simulink model "HIL_Testing_SW"  (Simulink 7.5)
settings: Solver=ode1  StartTime=0.0  StopTime=Inf  FixedStep=0.001  RelTol=1e-3
PostLoadFcn:
  | , if any(exist('dsrtsu_mdlpostloadfcn', 'file') == [2, 3, 6]), try dsrtsu_mdlpostloadfcn('Execute', bdroot); catch fprintf('Error in PostLoadFcn (dsrtsu_mdlpostloadfcn) for model "%s":\n %s\n', bdroot, lasterr); end, end,
undefined symbols (not defined in the file): CeBSER_Cnt_NumTempAxisPts, ChargeCord, ChargeCord_Control, ChargeToSOCCurr, ChrgCurrLim, CrntSens1Fine, CS_SOCSetPt, CyclerMaxChrgPwr, CyclerMaxDschrgPwr, deltaAhr, Drive_1, Drive_10, Drive_11, Drive_12, Drive_13, Drive_14, Drive_15, Drive_16, Drive_17, Drive_18, Drive_19, Drive_2, Drive_20, Drive_21, Drive_22, Drive_23, Drive_24, Drive_25, Drive_26, Drive_27, Drive_28, Drive_29, Drive_3, Drive_30, Drive_31, Drive_32, Drive_33, Drive_34, Drive_35, Drive_36, Drive_37, Drive_38, Drive_39, Drive_4, Drive_40, Drive_41, Drive_42, Drive_43, Drive_44, Drive_45, Drive_46, Drive_47, Drive_48, Drive_49, Drive_5, Drive_50, Drive_51, Drive_6, Drive_7, Drive_8 ... (+50)
libraries: simulink x129, rtican x50, rti2211sailib x5, rti2211serlib x5, rti2202miolib x3
(part 17 of 23)

== system HIL_Testing_SW/TX/Tx_Cycler/TX_ABC_ChB/msg_0x1A2_Upp_Lim_B_out ==
  Counter : Inport  OutDataType=sfix(16)  OutScaling=2^0
  Enable : EnablePort  StatesWhenEnabling=reset
  Constant1 : Constant  Value=1000  OutDataType=sfix(16)  OutScaling=2^0
  Data Store Read : DataStoreRead  DataStoreName=ChrgCurrLim  SampleTime=-1
  Data Store Read1 : DataStoreRead  DataStoreName=Voltage_Lid  SampleTime=-1
  Data Store Read2 : DataStoreRead  DataStoreName=CyclerMaxChrgPwr  SampleTime=-1
  Data Type Conversion : DataTypeConversion  OutDataTypeMode=double  OutDataType=fixdt(1, 16)  OutScaling=2^0  OutDataTypeStr=double
  Data Type Conversion1 : DataTypeConversion  OutDataTypeMode=double  OutDataType=fixdt(1, 16)  OutScaling=2^0  OutDataTypeStr=double
  Data Type Conversion{2..4,7} (4 alike) : DataTypeConversion  OutDataType=fixdt(1, 16)  OutScaling=2^0
  Product : Product  OutDataType=sfix(16)  OutScaling=2^0  RndMeth=Zero
  Terminator : Terminator
  Upp_Lim_B_out : rtican/RTICAN Transmit (TX)   SystemSampleTime=-1  Reserved1=[]  Reserved2=[]  Reserved3=[]  Reserved4=[]  SfcnMessage=[]  Msg_Struct=[]  BoardTypeNo=[]  BoardNo=[]  ChannelNo=[]  Parameters=[]  DialogFcn=[]  UnitName=[]  Revision=[]  UnitValues=[]  DSProperties=struct('RTI',struct('Version',uint32(5),'BlockType',struct('isSLSource',uint8(1),'isSLSink',uint8(1),'isHWSource',uint8(0),'isHWSink',uint8(0),'isSetup',uint8(0),'isInline',uint8(1),'isNonInline',uint8(0),'isInterrupt',uint8(0),'isChannelwise',uint8(0)),'IOBoardType','RTICAN','UnitType','MESSAGE','Identifier','TX','DialogType','MSVC','BlockSet','RTICAN','SlaveProcessor','CAN'))  RTIBlockInterface=struct('InputPortsWidth',int32([1 1 1 1]),'InputPortsActive',[1 1 1 1],'InputPortsName',{{'Upp_Powr_Lim_B_out','Counter_Stamp3_B','Upp_Curr_Lim_B_out','Upp_Volt_Lim_B_out'}},'InputPortsDataType',{{'SS_DOUBLE','SS_DOUBLE','SS_DOUBLE','SS_DOUBLE'}},'OutputPortsWidth',int32(1),'OutputPortsActive',1,'OutputPortsName',{{['TX status']}},'DialogFcn','rtican_message_interface_gui','BlockDisplay',{{'','center'}},'IconTransparency','on','InitLevel',3,'BlockName',struct('Token',{{'Upp_Lim_B_out'}}),'SampleTime',{{-1}},'TriggerPort',{{'none'}},'EnablePort',{{'none'}})  RTIBlockParameters=struct('BoardTypeNo',{{2211,'OFF',[]}},'BoardNo',{{2,'ON',[1 16]}},'ChannelNo',{{1,'ON',[1 2]}},'Parameters',{{struct('DataFileSupport',struct('DataFileSelectedMaster',1,'DataFileSelectedLocal',1,'DataFileName','c:\data\testing\av900_dbc\av900_mod.dbc|','DataFileDate',{{{['20-Apr-2011 08:23:37']}}},'SelectedFile','av900_dbc\av900_mod.dbc','InterfaceFcn','rtican_dbc_file_parser'),'Options',struct('StatusSelected',1,'TimeSelected',0,'DeltaTimeSelected',0,'DelayTimeSelected',0,'DelayTimeTXCommandSelected',0,'EncodeSetUnusedBitsToOne',0,'EnableMsgLoopback',0,'TriggerPort',struct('Selected',0,'TriggerType',0),'EnablePortSelected',0,'SignalOnPortnameSelected',1,'UserCoding',struct('Selected',0,'InterfaceFile','UserEncodingFile','FcnName','UserEncodeFcn','InportSelected',0,'InportWidth',1,'OutportSelected',0,'OutportWidth',1),'TerminationMsg',struct('Selected',0,'Byte0_7','0'),'InitialMsg',struct('Selected',0,'Byte0_7','0')),'Message',struct('MsgOnBlocknameSelected',1,'MsgName','Upp_Lim_B_out','MsgIdFormat',0,'MsgId',418,'MsgLength',7,'NumSignals',4,'SampleTime',-1,'StartTime',struct('Selected',0,'Value',0),'AutoRepeatTime',struct('Selected',0,'Value',0.1),'Timeout',struct('Selected',0,'Value',0.1),'DelayTime',struct('Selected',0,'Value',0.1),'Signal',struct('SgnName',{'Upp_Powr_Lim_B_out','Counter_Stamp3_B','Upp_Curr_Lim_B_out','Upp_Volt_Lim_B_out'},'SgnStartBit',{0,0,16,32},'SgnLength',{16,8,16,16},'SgnType',{0,0,0,0},'ModeValue',{-1,-1,-1,-1},'DataType',{1,0,1,1},'ByteLayout',{2,0,2,2},'Factor',{10,1,0.04,0.05},'Offset',{0,0,0,0},'SgnComment',{{''},{''},{''},{''}},'SgnUnit',{'W','code','A','V'},'Min',{-327680,0,-1310.72,-1638.4},'Max',{327670,255,1310.68,1638.35},'SLDataType',{'SS_DOUBLE','SS_DOUBLE','SS_DOUBLE','SS_DOUBLE'}),'MsgIdNumFormat',0,'MsgComment',{{''}}),'Version',1.2,'general',struct('isFromLib',0)),'OFF',[]}},'GroupId',{{struct('Group',{{'RTICAN'}},'No',6,'Behavior',{{'NAMECHANGE'}},'BlockType',{{'SINK'}},'NameChangeFlag',0),'OFF',[]}},'SFcnRTICANMessage',{{struct('MsgType','TX','SFcnPortType','Scalar','MsgName','Upp_Lim_B_out','MsgIdFormat','STD','MsgId',418,'MsgLength',7,'NumSignals',4,'SampleTime',-1,'StartTime',struct('Selected','no','Value',0),'AutoRepeatTime',struct('Selected','no','Value',0.1),'Timeout',struct('Selected','no','Value',0.1),'Signal',struct('SgnName',{'Upp_Powr_Lim_B_out','Counter_Stamp3_B','Upp_Curr_Lim_B_out','Upp_Volt_Lim_B_out'},'SgnStartBit',{0,0,16,32},'SgnLength',{16,8,16,16},'SgnType',{'standard','standard','standard','standard'},'ModeValue',{-1,-1,-1,-1},'DataType',{['signed int'],['unsigned int'],['signed int'],['signed int']},'ByteLayout',{['motorola back.'],['little endian'],['motorola back.'],['motorola back.']},'Factor',{10,1,0.04,0.05},'Offset',{0,0,0,0},'SLDataType',{'SS_DOUBLE','SS_DOUBLE','SS_DOUBLE','SS_DOUBLE'}),'StatusSelected','yes','TimeSelected','no','DeltaTimeSelected','no','DelayTimeSelected','no','DelayTimeTXCommandSelected','no','EncodeSetUnusedBitsToOne','no','EnableMsgLoopback','no','TriggerPort',struct('Selected','no','TriggerType',0),'EnablePortSelected','no','UserCoding',struct('Selected','no','InterfaceFile','UserEncodingFile','FcnName','UserEncodeFcn','InportSelected','no','InportWidth',1,'OutportSelected','no','OutportWidth',1),'TerminationMsg',struct('Selected','no','Byte0','0x00','Byte1','0x00','Byte2','0x00','Byte3','0x00','Byte4','0x00','Byte5','0x00','Byte6','0x00','Byte7','0x00'),'InitialMsg',struct('Selected','no','Byte0','0x00','Byte1','0x00','Byte2','0x00','Byte3','0x00','Byte4','0x00','Byte5','0x00','Byte6','0x00','Byte7','0x00'),'BoardType','DS2211','BoardNo',2,'ControllerNo',1),'OFF',[]}},'TLCFileName',{{'rtican_tx_message','OFF',[]}})  RTISFcnParameters=struct('SFcnRTICANMessage','struct','TLCFileName','char')  RTIBlockParaDefault=struct('BoardTypeNo',4302,'BoardNo',1,'ChannelNo',1,'Parameters',struct('DataFileSupport',struct('DataFileSelectedMaster',0,'DataFileSelectedLocal',0,'DataFileName','','DataFileDate','','SelectedFile',['<no file selected>']),'Options',struct('StatusSelected',1,'TimeSelected',1,'DeltaTimeSelected',1,'DelayTimeSelected',1,'DelayTimeTXCommandSelected',0,'EncodeSetUnusedBitsToOne',0,'EnableMsgLoopback',0,'TriggerPort',struct('Selected',0,'TriggerType','rising'),'EnablePortSelected',0,'SignalOnPortnameSelected',1,'UserCoding',struct('Selected',0,'InterfaceFile','UserEncodingFile','FcnName','UserEncodeFcn','InportSelected',0,'InportWidth',1,'OutportSelected',0,'OutportWidth',1),'TerminationMsg',struct('Selected',0,'Byte0_7','0'),'InitialMsg',struct('Selected',0,'Byte0_7','0')),'Message',struct('MsgOnBlocknameSelected',0,'MsgName',['TX Message'],'MsgIdFormat',0,'MsgId',100,'MsgLength',8,'NumSignals',1,'SampleTime',-1,'StartTime',struct('Selected',0,'Value',0),'AutoRepeatTime',struct('Selected',0,'Value',0.1),'Timeout',struct('Selected',0,'Value',0.1),'DelayTime',struct('Selected',0,'Value',0.1),'Signal',struct('SgnName',['TX signal'],'SgnStartBit',0,'SgnLength',8,'SgnType',0,'ModeValue',-1,'DataType',0,'SLDataType','SS_DOUBLE','ByteLayout',0,'Factor',1,'Offset',0,'Min',0,'Max',255,'SgnComment',{{}},'SgnUnit',''),'MsgIdNumFormat',0,'MsgComment',{{''}}),'Version',1.2,'general',struct('isFromLib',1)),'GroupId',struct('Group',{{'RTICAN'}},'No',1,'Behavior',{{'NAMECHANGE'}},'BlockType',{{'SINK'}},'NameChangeFlag',0),'SFcnRTICANMessage',struct('MsgType','TX','MsgName',['TX Message'],'MsgIdFormat','STD','MsgId',100,'MsgLength',2,'NumSignals',1,'SampleTime',-1,'StartTime',struct('Selected','no','Value',0),'AutoRepeatTime',struct('Selected','no','Value',0.1),'Timeout',struct('Selected','no','Value',0.1),'DelayTime',struct('Selected','no','Value',0.1),'Signal',struct('SgnName',['TX signal'],'SgnStartBit',0,'SgnLength',8,'SgnType','standard','ModeValue',-1,'DataType',['unsigned int'],'ByteLayout',['little endian'],'SLDataType','SS_DOUBLE','Factor',1,'Offset',0),'StatusSelected','yes','TimeSelected','yes','DeltaTimeSelected','yes','DelayTimeSelected','yes','EnablePortSelected','no','EnableMsgLoopback','no','DelayTimeTXCommandSelected','no','EncodeSetUnusedBitsToOne','no','UserCoding',struct('Selected','no','InterfaceFile','UserDecodingFile','FcnName','UserDecodeFcn','InportSelected','no','InportWidth',1,'OutportSelected','no','OutportWidth',1),'TerminationMsg',struct('Selected','no','Byte0','0x00','Byte1','0x00','Byte2','0x00','Byte3','0x00','Byte4','0x00','Byte5','0x00','Byte6','0x00','Byte7','0x00'),'InitialMsg',struct('Selected','no','Byte0','0x00','Byte1','0x00','Byte2','0x00','Byte3','0x00','Byte4','0x00','Byte5','0x00','Byte6','0x00','Byte7','0x00'),'TriggerPort',struct('Selected','no','TriggerType','rising'),'BoardType','DS4302','BoardNo',1,'ControllerNo',1,'SFcnPortType','Scalar'),'TLCFileName','rtican_tx_message')
      settings: AttributesFormatString=Group Id: RTICAN6\n
  wires:
  Data Store Read/1 -> Data Type Conversion/1
  Data Store Read1/1 -> Data Type Conversion1/1
  Data Store Read2/1 -> Product/1
  Constant1/1 -> Product/2
  Upp_Lim_B_out/1 -> Terminator/1
  Data Type Conversion1/1 -> Data Type Conversion4/1
  Data Type Conversion/1 -> Data Type Conversion3/1
  Counter/1 -> Data Type Conversion2/1
  Product/1 -> Data Type Conversion7/1
  Data Type Conversion7/1 -> Upp_Lim_B_out/1
  Data Type Conversion2/1 -> Upp_Lim_B_out/2
  Data Type Conversion3/1 -> Upp_Lim_B_out/3
  Data Type Conversion4/1 -> Upp_Lim_B_out/4

== system HIL_Testing_SW/HWO/TX HVEM/ChargeCord_Control/Cord Connected/110 Connected ==
  note: Updated to 108 cals for Ofst and Slp
  Volt_in : Inport  OutDataType=sfix(16)  OutScaling=2^0
  Current_in : Inport  Port=2  OutDataType=sfix(16)  OutScaling=2^0
  Temp_in : Inport  Port=3  OutDataType=sfix(16)  OutScaling=2^0
  DC_in : Inport  Port=4  OutDataType=sfix(16)  OutScaling=2^0
  Action Port : ActionPort  ActionType=then
  110_Volts : Constant  Value=110  OutDataType=sfix(16)  OutScaling=2^0  OutDataTypeStr=Inherit: Inherit via back propagation
  Fcn : Fcn  Expr=((u(1)-32.5)/2.75)
  Volt_out : Outport  OutDataType=sfix(16)  OutScaling=2^0
  Current_out : Outport  Port=2  OutDataType=sfix(16)  OutScaling=2^0
  Temp_out : Outport  Port=3  OutDataType=sfix(16)  OutScaling=2^0
  DC_Out : Outport  Port=4  OutDataType=sfix(16)  OutScaling=2^0
  PrcsdVolt_DC : Outport  Port=5  OutDataType=sfix(16)  OutScaling=2^0
  wires:
  DC_in/1 -> DC_Out/1
  Temp_in/1 -> Temp_out/1
  Current_in/1 -> Current_out/1
  Fcn/1 -> PrcsdVolt_DC/1
  Volt_in/1 -> Volt_out/1
  110_Volts/1 -> Fcn/1

== system HIL_Testing_SW/HWO/TX HVEM/ChargeCord_Control/Cord Connected/220 Connected ==
  note: Updated to 108 cals for Ofst and Slp
  Volt_in : Inport  OutDataType=sfix(16)  OutScaling=2^0
  Current_in : Inport  Port=2  OutDataType=sfix(16)  OutScaling=2^0
  Temp_in : Inport  Port=3  OutDataType=sfix(16)  OutScaling=2^0
  DC_in : Inport  Port=4  OutDataType=sfix(16)  OutScaling=2^0
  Action Port : ActionPort  ActionType=elseif
  220_Volts : Constant  Value=220  OutDataType=sfix(16)  OutScaling=2^0  OutDataTypeStr=Inherit: Inherit via back propagation
  Fcn : Fcn  Expr=((u(1)-32.5)/2.75)
  Volt_out : Outport  OutDataType=sfix(16)  OutScaling=2^0
  Current_out : Outport  Port=2  OutDataType=sfix(16)  OutScaling=2^0
  Temp_out : Outport  Port=3  OutDataType=sfix(16)  OutScaling=2^0
  DC_Out : Outport  Port=4  OutDataType=sfix(16)  OutScaling=2^0
  PrcsdVolt_DC : Outport  Port=5  OutDataType=sfix(16)  OutScaling=2^0
  wires:
  Volt_in/1 -> Volt_out/1
  Current_in/1 -> Current_out/1
  Temp_in/1 -> Temp_out/1
  DC_in/1 -> DC_Out/1
  Fcn/1 -> PrcsdVolt_DC/1
  220_Volts/1 -> Fcn/1

== system HIL_Testing_SW/HWO/TX HVEM/ChargeCord_Control/Cord Connected/AC Enabled ==
  Volt_in : Inport  OutDataType=sfix(16)  OutScaling=2^0
  Current_in : Inport  Port=2  OutDataType=sfix(16)  OutScaling=2^0
  Action Port : ActionPort  ActionType=then
  Volt_out : Outport  OutDataType=sfix(16)  OutScaling=2^0
  Current_out : Outport  Port=2  OutDataType=sfix(16)  OutScaling=2^0
  wires:
  Current_in/1 -> Current_out/1
  Volt_in/1 -> Volt_out/1

== system HIL_Testing_SW/HWO/TX HVEM/ChargeCord_Control/Cord Connected/AC Not Enabled ==
  Volt_in : Inport  OutDataType=sfix(16)  OutScaling=2^0
  Current_in : Inport  Port=2  OutDataType=sfix(16)  OutScaling=2^0
  Action Port : ActionPort  ActionType=else
  Volt_out : Outport  OutDataType=sfix(16)  OutScaling=2^0
  Current_out : Outport  Port=2  OutDataType=sfix(16)  OutScaling=2^0
  wires:
  Volt_in/1 -> Volt_out/1
  Current_in/1 -> Current_out/1

== system HIL_Testing_SW/HWO/TX HVEM/ChargeCord_Control/Cord Connected/Not Connected ==
  Volt_in : Inport  OutDataType=sfix(16)  OutScaling=2^0
  Current_in : Inport  Port=2  OutDataType=sfix(16)  OutScaling=2^0
  Temp_in : Inport  Port=3  OutDataType=sfix(16)  OutScaling=2^0
  DC_in : Inport  Port=4  OutDataType=sfix(16)  OutScaling=2^0
  Action Port : ActionPort  ActionType=else
  NotConnected_Volts : Constant  Value=100  OutDataType=sfix(16)  OutScaling=2^0  OutDataTypeStr=Inherit: Inherit via back propagation
  Volt_out : Outport  OutDataType=sfix(16)  OutScaling=2^0
  Current_out : Outport  Port=2  OutDataType=sfix(16)  OutScaling=2^0
  Temp_out : Outport  Port=3  OutDataType=sfix(16)  OutScaling=2^0
  DC_Out : Outport  Port=4  OutDataType=sfix(16)  OutScaling=2^0
  PrcsdVolt_DC : Outport  Port=5  OutDataType=sfix(16)  OutScaling=2^0
  wires:
  Volt_in/1 -> Volt_out/1
  Current_in/1 -> Current_out/1
  Temp_in/1 -> Temp_out/1
  DC_in/1 -> DC_Out/1
  NotConnected_Volts/1 -> PrcsdVolt_DC/1

== system HIL_Testing_SW/LionsHeart/FeaturePresentation/Down_to_Business/DriveProfile_ModeControl/Capacity Test ==
  Current_Cntrl : Inport  OutDataType=fixdt(1, 16)  OutScaling=2^0
  Voltage_Cntrl : Inport  Port=2  OutDataType=fixdt(1, 16)  OutScaling=2^0
  MaxCall_PackVolt : Inport  Port=3  OutDataType=fixdt(1, 16)  OutScaling=2^0
  MinCall_PackVolt : Inport  Port=4  OutDataType=fixdt(1, 16)  OutScaling=2^0
  CyclerVoltage : Inport  Port=5  OutDataType=fixdt(1, 16)  OutScaling=2^0
  Enable : EnablePort  StatesWhenEnabling=reset
  Capacity_Test : Stateflow chart  TreatAsAtomicUnit=on
  Data Store Read : DataStoreRead  DataStoreName=Voltage_Floor  SampleTime=0
  Data Store Read1 : DataStoreRead  DataStoreName=Voltage_Lid  SampleTime=0
  Data Store Read10 : DataStoreRead  DataStoreName=DschrgCurrLim  SampleTime=0
  Data Store Read11 : DataStoreRead  DataStoreName=CapCycles  SampleTime=0
  Data Store Read12 : DataStoreRead  DataStoreName=CapRestTime  SampleTime=0
  Data Store Read13 : DataStoreRead  DataStoreName=OCV_Zero  SampleTime=0
  Data Store Read2 : DataStoreRead  DataStoreName=TerminationCurrent  SampleTime=0
  Data Store Read3 : DataStoreRead  DataStoreName=Voltage_Floor_Cell  SampleTime=0
  Data Store Read4 : DataStoreRead  DataStoreName=C_Rate  SampleTime=0
  Data Store Read5 : DataStoreRead  DataStoreName=Voltage_Lid_Cell  SampleTime=0
  Data Store Read6 : DataStoreRead  DataStoreName=RateFactor  SampleTime=0
  Data Store Read7 : DataStoreRead  DataStoreName=MaxCell_Enbl  SampleTime=0
  Data Store Read8 : DataStoreRead  DataStoreName=MinCell_Enbl  SampleTime=0
  Data Store Read9 : DataStoreRead  DataStoreName=ChrgCurrLim  SampleTime=0
  Data Store Write1 : DataStoreWrite  DataStoreName=ChrgCurrLim  SampleTime=-1
  Data Store Write2 : DataStoreWrite  DataStoreName=DschrgCurrLim  SampleTime=-1
  Data Store Write3 : DataStoreWrite  DataStoreName=ContactorOverride  SampleTime=-1
  Data Type Conversion : DataTypeConversion  OutDataTypeMode=single  OutDataType=sfix(16)  OutScaling=2^0  OutDataTypeStr=single
  Data Type Conversion1 : DataTypeConversion  OutDataTypeMode=single  OutDataType=sfix(16)  OutScaling=2^0  OutDataTypeStr=single
  Gain : Gain  ParameterDataType=fixdt(1, 16)  ParameterScaling=2^0  OutDataType=fixdt(1, 16)  OutScaling=2^0
  Terminator1 : Terminator
  Terminator2 : Terminator
  Terminator4 : Terminator
  simstep : Constant  Tag=R12-1  Value=SimStep_dT  OutDataTypeMode=double  OutDataType=sfix(16)  OutScaling=2^0  OutDataTypeStr=double
  Profile_Data_cap : Outport  OutDataType=sfix(16)  OutScaling=2^0
  Mode_Cntrl_cap : Outport  Port=2  OutDataType=sfix(16)  OutScaling=2^0
  CapStep : Outport  Port=3  OutDataType=sfix(16)  OutScaling=2^0
  ResetSOCFlg : Outport  Port=4  OutDataType=sfix(16)  OutScaling=2^0
  wires:
  Current_Cntrl/1 -> [Current_Cntrl]
  Voltage_Cntrl/1 -> [Voltage_Cntrl]
  simstep/1 -> Data Type Conversion1/1
  Data Type Conversion/1 -> Profile_Data_cap/1
  Capacity_Test/1(Control_Value_cap) -> Data Type Conversion/1
  Data Type Conversion1/1 -> Capacity_Test/7(sim_step_time)
  Capacity_Test/2(WaitTime) -> Terminator2/1  "Waitime"
  Capacity_Test/4(cycle) -> Terminator4/1  "cycle"
  Data Store Read9/1 -> Capacity_Test/9(ChrgCurrLim)
  Data Store Read10/1 -> Capacity_Test/10(DischrgCurrLim)
  Capacity_Test/5(DischrgCurrLim_Tmp) -> Data Store Write2/1
  Capacity_Test/6(ChrgCurrLim_Tmp) -> Data Store Write1/1
  Capacity_Test/7(Step) -> CapStep/1
  MaxCall_PackVolt/1 -> [MaxCell_PackVolt]
  MinCall_PackVolt/1 -> [MinCell_PackVolt]
  [MinCell_PackVolt] -> Capacity_Test/11(PackVolt_MinCell)
  [MaxCell_PackVolt] -> Capacity_Test/12(PackVolt_MaxCell)
  Data Store Read6/1 -> Capacity_Test/13(RateFactor)
  Capacity_Test/3(Mode_Cntrl_cap) -> Mode_Cntrl_cap/1
  Data Store Read3/1 -> Capacity_Test/14(Vfloor_cell)
  Data Store Read5/1 -> Capacity_Test/15(Vlid_cell)
  Data Store Read7/1 -> Capacity_Test/16(MaxCell_Enbl)
  Data Store Read8/1 -> Capacity_Test/17(MinCell_Enbl)
  CyclerVoltage/1 -> [CyclerVoltage]
  [CyclerVoltage] -> Capacity_Test/18(CyclerVoltage)
  Data Store Read11/1 -> Capacity_Test/6(NumberCycles)
  Data Store Read12/1 -> Capacity_Test/8(RestTime)
  Data Store Read4/1 -> Capacity_Test/20(CRate)
  [Voltage_Cntrl] -> Capacity_Test/4(Voltage_Cntrl)
  [Current_Cntrl] -> Capacity_Test/5(Current_Cntrl)
  Data Store Read1/1 -> Capacity_Test/2(Vlid)
  Data Store Read2/1 -> Capacity_Test/3(CurrentTerm)
  Data Store Read13/1 -> Capacity_Test/19(OCV_Zero)
  Capacity_Test/8(ContactorOverride) -> Data Store Write3/1
  Gain/1 -> Terminator1/1  "Cappy2"
  Capacity_Test/9(Cappy) -> Gain/1  "Cappy"
  Data Store Read/1 -> Capacity_Test/1(Vfloor)
  Capacity_Test/10(ResetSOCFlg) -> ResetSOCFlg/1  "ResetSOCFlg"

== system HIL_Testing_SW/LionsHeart/FeaturePresentation/Down_to_Business/DriveProfile_ModeControl/Charging_Mode ==
  note: Select Current for Charge
  Current : Inport  OutDataType=fixdt(1, 16)  OutScaling=2^0
  Voltage : Inport  Port=2  OutDataType=fixdt(1, 16)  OutScaling=2^0
  ChargeCurrSelect : Inport  Port=3  OutDataType=fixdt(1, 16)  OutScaling=2^0
  SOCTarget : Inport  Port=4  OutDataType=fixdt(1, 16)  OutScaling=2^0
  PackVolt_MaxCell : Inport  Port=5  OutDataType=fixdt(1, 16)  OutScaling=2^0
  PackVolt_MinCell : Inport  Port=6  OutDataType=fixdt(1, 16)  OutScaling=2^0
  SOC : Inport  Port=7  OutDataType=fixdt(1, 16)  OutScaling=2^0
  Voltage_Cntrl : Inport  Port=8  OutDataType=fixdt(1, 16)  OutScaling=2^0
  Current_Cntrl : Inport  Port=9  OutDataType=fixdt(1, 16)  OutScaling=2^0
  Enable : EnablePort  StatesWhenEnabling=reset
  Charge Selector : MultiPortSwitch  DataPortOrder=Zero-based contiguous  zeroidx=on  OutDataType=sfix(16)  OutScaling=2^0
  Charging Logic1 : Stateflow chart  TreatAsAtomicUnit=on
  Data Store Read : DataStoreRead  DataStoreName=VoltageTerm  SampleTime=0
  Data Store Read1 : DataStoreRead  DataStoreName=TerminationCurrent  SampleTime=0
  Data Store Read10 : DataStoreRead  DataStoreName=DschrgCurrLim  SampleTime=0
  Data Store Read11 : DataStoreRead  DataStoreName=RateFactor  SampleTime=0
  Data Store Read12 : DataStoreRead  DataStoreName=Voltage_Floor  SampleTime=0
  Data Store Read13 : DataStoreRead  DataStoreName=CyclerOffset  SampleTime=0
  Data Store Read15 : DataStoreRead  DataStoreName=ChargeToSOCRate  SampleTime=0
  Data Store Read2 : DataStoreRead  DataStoreName=WaitTime  SampleTime=0
  Data Store Read3 : DataStoreRead  DataStoreName=Voltage_Lid  SampleTime=0
  Data Store Read4 : DataStoreRead  DataStoreName=MaxCell_Enbl  SampleTime=0
  Data Store Read5 : DataStoreRead  DataStoreName=VoltageTerm_MaxCell  SampleTime=0
  Data Store Read6 : DataStoreRead  DataStoreName=TwoTwentyChrgCurr  SampleTime=0
  Data Store Read7 : DataStoreRead  DataStoreName=OneTenChargeCurr  SampleTime=0
  Data Store Read8 : DataStoreRead  DataStoreName=MinCell_Enbl  SampleTime=0
  Data Store Read9 : DataStoreRead  DataStoreName=ChrgCurrLim  SampleTime=0
  Data Store Write15 : DataStoreWrite  DataStoreName=ChrgCurrLim  SampleTime=-1
  Data Store Write16 : DataStoreWrite  DataStoreName=DschrgCurrLim  SampleTime=-1
  Data Type Conversion : DataTypeConversion  OutDataTypeMode=single  OutDataType=sfix(16)  OutScaling=2^0  OutDataTypeStr=single
  Data Type Conversion1 : DataTypeConversion  OutDataTypeMode=single  OutDataType=sfix(16)  OutScaling=2^0  OutDataTypeStr=single
  Terminator : Terminator
  simstep : Constant  Tag=R12-1  Value=SimStep_dT  OutDataTypeMode=double  OutDataType=sfix(16)  OutScaling=2^0  OutDataTypeStr=double
  Profile_Data_chrg : Outport  OutDataType=sfix(16)  OutScaling=2^0
  Mode_Cntrl_chrg : Outport  Port=2  OutDataType=sfix(16)  OutScaling=2^0
  ChargeStep : Outport  Port=3  OutDataType=sfix(16)  OutScaling=2^0
  wires:
  Charge Selector/1 -> [ChargeCurrent]
  Current/1 -> [CyclerCurrent]
  Voltage/1 -> [Voltage]
  [ChargeCurrent] -> Charging Logic1/1(RateChrg)
  simstep/1 -> Data Type Conversion1/1
  Data Type Conversion1/1 -> Charging Logic1/5(sim_step_time)
  Data Store Read2/1 -> Charging Logic1/6(WaitTime1)
  SOC/1 -> Charging Logic1/8(SOC)
  [ChargeCurrSelect] -> Charging Logic1/7(ChargeSelect)
  Charging Logic1/3(Mode_Cntrl_cap) -> Mode_Cntrl_chrg/1
  Charging Logic1/1(Control_Value_cap) -> Data Type Conversion/1
  Charging Logic1/2(WaitTime) -> Terminator/1
  Data Store Read1/1 -> Charging Logic1/3(CurrentTerm)
  Data Store Read3/1 -> Charging Logic1/9(VoltageLid)
  Data Store Read6/1 -> Charge Selector/3
  Data Store Read7/1 -> Charge Selector/2
  Charging Logic1/4(ChargeLimit_Temp) -> Data Store Write15/1
  Charging Logic1/5(DisChrgCurr_Limit) -> Data Store Write16/1
  Data Store Read9/1 -> Charging Logic1/10(ChargeLimitCal)
  Data Store Read10/1 -> Charging Logic1/11(DisChrgCurrLimit_Cal)
  Charging Logic1/6(Step) -> ChargeStep/1
  ChargeCurrSelect/1 -> [ChargeCurrSelect]
  [ChargeCurrSelect] -> Charge Selector/1
  [Current_Cntrl] -> Charging Logic1/4(Current_Cntrl)
  [Voltage] -> Charging Logic1/12(CyclerVoltage)
  Data Store Read11/1 -> Charging Logic1/14(RateFactor)
  Data Type Conversion/1 -> Profile_Data_chrg/1
  [SOCTarget] -> Charging Logic1/13(SOCTarget)
  Data Store Read/1 -> Charging Logic1/2(VoltageSetPoint)
  SOCTarget/1 -> [SOCTarget]
  Data Store Read12/1 -> Charging Logic1/15(VFloor)
  PackVolt_MaxCell/1 -> [PackVoltage_MaxCell]
  PackVolt_MinCell/1 -> [PackVoltage_MinCell]
  [PackVoltage_MaxCell] -> Charging Logic1/16(PackVoltage_MaxCell)
  [PackVoltage_MinCell] -> Charging Logic1/17(PackVoltage_MinCell)
  Data Store Read5/1 -> Charging Logic1/18(VoltageSetPt_Max)
  Data Store Read15/1 -> Charge Selector/4
  Data Store Read4/1 -> Charging Logic1/20(MaxCell_Enbl)
  Data Store Read8/1 -> Charging Logic1/21(MinCell_Enbl)
  Voltage_Cntrl/1 -> [Voltage_Cntrl]
  Current_Cntrl/1 -> [Current_Cntrl]
  [Voltage_Cntrl] -> Charging Logic1/19(Voltage_Cntrl)
  Data Store Read13/1 -> Charging Logic1/22(CyclerOffset)

== system HIL_Testing_SW/LionsHeart/FeaturePresentation/Down_to_Business/DriveProfile_ModeControl/Drive_Profile ==
  note: Mode_Cntrl:
      | ****************
      | 0 = Voltage
      | 1 = Current
      | 2 = Power
      | 3 = Standby
  cycle_enable : Inport  OutDataType=sfix(16)  OutScaling=2^0
  SOC : Inport  Port=2  OutDataType=sfix(16)  OutScaling=2^0
  Current : Inport  Port=3  OutDataType=fixdt(1, 16)  OutScaling=2^0
  Voltage : Inport  Port=4  OutDataType=fixdt(1, 16)  OutScaling=2^0
  BatTemp : Inport  Port=5  OutDataType=fixdt(1, 16)  OutScaling=2^0
  PowerCycle : Inport  Port=6  OutDataType=sfix(16)  OutScaling=2^0
  CSSwitch : Inport  Port=7  OutDataType=sfix(16)  OutScaling=2^0
  StartTime : Inport  Port=8  OutDataType=sfix(16)  OutScaling=2^0
  EndTime : Inport  Port=9  OutDataType=sfix(16)  OutScaling=2^0
  Enable : EnablePort  StatesWhenEnabling=reset
  CD : Subsystem
  Data Type Conversion1 : DataTypeConversion  OutDataTypeMode=boolean  OutDataType=sfix(16)  OutScaling=2^0  OutDataTypeStr=boolean
  PowerMode : Constant  Value=single(2)  OutDataType=sfix(16)  OutScaling=2^0
  Relational Operator : RelationalOperator  LogicOutDataTypeMode=boolean  OutDataTypeStr=boolean
  Standby : Constant  Value=single(3)  OutDataType=sfix(16)  OutScaling=2^0
  Switch : Switch  Threshold=.5  OutDataType=sfix(16)  OutScaling=2^0
  Profile_Data_drive : Outport  OutDataType=sfix(16)  OutScaling=2^0
  Mode_Cntrl_drive : Outport  Port=2  OutDataType=sfix(16)  OutScaling=2^0
  ProfileEndTime : Outport  Port=3  OutDataType=sfix(16)  OutScaling=2^0
  LoopTime : Outport  Port=4  OutDataType=sfix(16)  OutScaling=2^0
  wires:
  SOC/1 -> [SOC]
  BatTemp/1 -> [BatTemp]
  Voltage/1 -> [Voltage]
  Current/1 -> [Current]
  cycle_enable/1 -> Data Type Conversion1/1
  PowerCycle/1 -> [Power_Cycle]
  PowerMode/1 -> Switch/3
  Switch/1 -> Mode_Cntrl_drive/1
  [Loop_Time] -> Relational Operator/1
  [ProfileEndTime] -> Relational Operator/2
  Relational Operator/1 -> Switch/2
  Standby/1 -> Switch/1
  CSSwitch/1 -> [SwitchMode]
  CD/2(LoopTime) -> [Loop_TimeCD]
  CD/1(ProfileTrigger) -> [ProfileData_PowerCD]
  [Power_Cycle] -> CD/1(PowercyleSelect)
  CD/3(ProfileEndTime) -> [ProfileEndTimeCD]
  Data Type Conversion1/1 -> [CycleEnable]
  [CycleEnable] -> CD/2(cycleEnbl)
  [ProfileData_PowerCD] -> Profile_Data_drive/1
  [Loop_TimeCD] -> LoopTime/1, [Loop_Time]
  [ProfileEndTimeCD] -> ProfileEndTime/1, [ProfileEndTime]
  StartTime/1 -> CD/3(StartTime)
  EndTime/1 -> CD/4(EndTime)

== system HIL_Testing_SW/LionsHeart/FeaturePresentation/Down_to_Business/DriveProfile_ModeControl/HPPC Test ==
  Current : Inport  OutDataType=fixdt(1, 16)  OutScaling=2^0
  Voltage : Inport  Port=2  OutDataType=fixdt(1, 16)  OutScaling=2^0
  Enable : EnablePort  StatesWhenEnabling=reset
  BeforeTime : Constant  Value=60  OutDataTypeMode=single  OutDataType=fixdt(1, 16)  OutScaling=2^0  OutDataTypeStr=single
  BtwnTime : Constant  Value=40  OutDataTypeMode=single  OutDataType=fixdt(1, 16)  OutScaling=2^0  OutDataTypeStr=single
  ChargeRate : Constant  OutDataTypeMode=single  OutDataType=fixdt(1, 16)  OutScaling=2^0  OutDataTypeStr=single
  Data Store Read : DataStoreRead  DataStoreName=VoltageTerm  SampleTime=0
  Data Store Read1 : DataStoreRead  DataStoreName=Voltage_Floor  SampleTime=0
  Data Store Read2 : DataStoreRead  DataStoreName=TerminationCurrent  SampleTime=0
  Data Store Read4 : DataStoreRead  DataStoreName=PackCapacity  SampleTime=0
  Data Store Read9 : DataStoreRead  DataStoreName=ChrgCurrLim  SampleTime=0
  Data Store Write15 : DataStoreWrite  DataStoreName=ChrgCurrLim  SampleTime=-1
  Data Type Conversion : DataTypeConversion  OutDataTypeMode=single  OutDataType=sfix(16)  OutScaling=2^0  OutDataTypeStr=single
  Data Type Conversion4 : DataTypeConversion  OutDataTypeMode=single  OutDataType=sfix(16)  OutScaling=2^0  OutDataTypeStr=single
  DischrgRate : Constant  Value=-1  OutDataTypeMode=single  OutDataType=fixdt(1, 16)  OutScaling=2^0  OutDataTypeStr=single
  FirstDischgTime : Constant  Value=150  OutDataTypeMode=single  OutDataType=fixdt(1, 16)  OutScaling=2^0  OutDataTypeStr=single
  HPPC_Test : Stateflow chart  TreatAsAtomicUnit=on
  PlchgCurr : Constant  Value=225  OutDataTypeMode=single  OutDataType=fixdt(1, 16)  OutScaling=2^0  OutDataTypeStr=single
  PldschgCurr : Constant  Value=-400  OutDataTypeMode=single  OutDataType=fixdt(1, 16)  OutScaling=2^0  OutDataTypeStr=single
  Product2 : Product  OutDataType=fixdt(1, 16)  OutScaling=2^0  RndMeth=Zero
  Product3 : Product  OutDataType=fixdt(1, 16)  OutScaling=2^0  RndMeth=Zero
  PulseTime : Constant  Value=10  OutDataTypeMode=single  OutDataType=fixdt(1, 16)  OutScaling=2^0  OutDataTypeStr=single
  RemDschgTime : Constant  Value=150  OutDataTypeMode=single  OutDataType=fixdt(1, 16)  OutScaling=2^0  OutDataTypeStr=single
  Rest : Constant  Value=7200  OutDataTypeMode=single  OutDataType=fixdt(1, 16)  OutScaling=2^0  OutDataTypeStr=single
  RestLong : Constant  Value=18000  OutDataTypeMode=single  OutDataType=fixdt(1, 16)  OutScaling=2^0  OutDataTypeStr=single
  RestShort : Constant  Value=60  OutDataTypeMode=single  OutDataType=fixdt(1, 16)  OutScaling=2^0  OutDataTypeStr=single
  Terminator : Terminator
  simstep : Constant  Tag=R12-1  Value=SimStep_dT  OutDataTypeMode=double  OutDataType=sfix(16)  OutScaling=2^0  OutDataTypeStr=double
  Mode_Cntrl_HPPC : Outport  OutDataType=sfix(16)  OutScaling=2^0
  Profile_Data_HPPC : Outport  Port=2  OutDataType=sfix(16)  OutScaling=2^0
  wires:
  Current/1 -> [Current]
  Voltage/1 -> [Voltage]
  ChargeRate/1 -> Product2/1
  Data Store Read4/1 -> Product2/2, Product3/2
  Product2/1 -> [ChrgRate]
  DischrgRate/1 -> Product3/1
  Product3/1 -> [DischrgRate]
  [DischrgRate] -> HPPC_Test/1(RateDischrg)
  [ChrgRate] -> HPPC_Test/2(RateChrg)
  Data Store Read/1 -> HPPC_Test/3(VoltageTerm)
  Data Store Read2/1 -> HPPC_Test/4(CurrentTerm)
  [Voltage] -> HPPC_Test/5(Voltage)
  [Current] -> HPPC_Test/6(Current)
  Data Store Read1/1 -> HPPC_Test/18(VoltageFloor)
  simstep/1 -> Data Type Conversion4/1
  Data Type Conversion4/1 -> HPPC_Test/8(sim_step_time)
  HPPC_Test/2(Mode_Cntrl) -> Mode_Cntrl_HPPC/1
  HPPC_Test/1(Control_Value) -> Data Type Conversion/1
  Data Type Conversion/1 -> Profile_Data_HPPC/1
  RestShort/1 -> HPPC_Test/7(RestShortSet)
  RestLong/1 -> HPPC_Test/9(LongRestSet)
  Rest/1 -> HPPC_Test/10(RestTimeSet)
  PulseTime/1 -> HPPC_Test/12(PulseTimeSet)
  BtwnTime/1 -> HPPC_Test/13(BtwnTimeSet)
  BeforeTime/1 -> HPPC_Test/15(RestBeforeSet)
  FirstDischgTime/1 -> HPPC_Test/16(DischrgTime)
  RemDschgTime/1 -> HPPC_Test/17(DischrgTime2)
  PldschgCurr/1 -> HPPC_Test/11(DischrgPulseCurr)
  PlchgCurr/1 -> HPPC_Test/14(ChrgPulseCurr)
  HPPC_Test/3(Step) -> Terminator/1
  Data Store Read9/1 -> HPPC_Test/19(ChrgCurrLim)
  HPPC_Test/4(ChrgCurrLim_Tmp) -> Data Store Write15/1

== system HIL_Testing_SW/LionsHeart/FeaturePresentation/Down_to_Business/DriveProfile_ModeControl/Idle ==
  TimeRequest : Inport  OutDataType=fixdt(1, 16)  OutScaling=2^0
  PowerReq : Inport  Port=2  OutDataType=fixdt(1, 16)  OutScaling=2^0
  CurrentReq : Inport  Port=3  OutDataType=fixdt(1, 16)  OutScaling=2^0
  Idle_Type : Inport  Port=4  OutDataType=fixdt(1, 16)  OutScaling=2^0
  Enable : EnablePort  StatesWhenEnabling=reset
  CurrentRequest : Constant  Value=-1  OutDataTypeMode=single  OutDataType=fixdt(1, 16)  OutScaling=2^0  OutDataTypeStr=single
  Data Store Read9 : DataStoreRead  DataStoreName=ManualIdle  SampleTime=0
  Data Type Conversion1 : DataTypeConversion  OutDataTypeMode=single  OutDataType=sfix(16)  OutScaling=2^0  OutDataTypeStr=single
  Idle : Stateflow chart  TreatAsAtomicUnit=on
  ManualIdle1 : Switch  Threshold=0.5  OutDataType=fixdt(1, 16)  OutScaling=2^0
  ManualIdle2 : Switch  Threshold=0.5  OutDataType=fixdt(1, 16)  OutScaling=2^0
  PowerRequest : Constant  Value=-4  OutDataTypeMode=single  OutDataType=fixdt(1, 16)  OutScaling=2^0  OutDataTypeStr=single
  simstep : Constant  Tag=R12-1  Value=SimStep_dT  OutDataTypeMode=double  OutDataType=sfix(16)  OutScaling=2^0  OutDataTypeStr=double
  Profile_Data_idle : Outport  OutDataType=sfix(16)  OutScaling=2^0
  Mode_Cntrl_idle : Outport  Port=2  OutDataType=sfix(16)  OutScaling=2^0
  IdleStep : Outport  Port=3  OutDataType=sfix(16)  OutScaling=2^0
  wires:
  simstep/1 -> Data Type Conversion1/1
  Data Type Conversion1/1 -> Idle/4(sim_step_time)
  TimeRequest/1 -> Idle/3(TimeRequest)
  Idle/1(Control_Value) -> Profile_Data_idle/1
  Idle/2(Mode_Cntrl) -> Mode_Cntrl_idle/1
  Idle/3(Step) -> IdleStep/1
  PowerRequest/1 -> ManualIdle1/1
  PowerReq/1 -> ManualIdle1/3
  Data Store Read9/1 -> ManualIdle1/2, ManualIdle2/2
  ManualIdle1/1 -> Idle/1(PowerRequest)
  CurrentRequest/1 -> ManualIdle2/1
  CurrentReq/1 -> ManualIdle2/3
  Idle_Type/1 -> Idle/5(Idle_Type)
  ManualIdle2/1 -> Idle/2(CurrentRequest)

== system HIL_Testing_SW/LionsHeart/FeaturePresentation/Down_to_Business/DriveProfile_ModeControl/Increment ==
  Voltage : Inport  OutDataType=fixdt(1, 16)  OutScaling=2^0
  PackVolt_MinCell : Inport  Port=2  OutDataType=fixdt(1, 16)  OutScaling=2^0
  Enable : EnablePort  StatesWhenEnabling=reset
  Data Store Read1 : DataStoreRead  DataStoreName=Pulse  SampleTime=0
  Data Store Read10 : DataStoreRead  DataStoreName=DschrgCurrLim  SampleTime=0
  Data Store Read2 : DataStoreRead  DataStoreName=Increment  SampleTime=0
  Data Store Read3 : DataStoreRead  DataStoreName=deltaAhr  SampleTime=0
  Data Store Read4 : DataStoreRead  DataStoreName=Ahr  SampleTime=0
  Data Store Read5 : DataStoreRead  DataStoreName=Voltage_Floor  SampleTime=0
  Data Store Read6 : DataStoreRead  DataStoreName=Voltage_Floor_Cell  SampleTime=0
  Data Store Write1 : DataStoreWrite  DataStoreName=DschrgCurrLim  SampleTime=-1
  Data Type Conversion1 : DataTypeConversion  OutDataTypeMode=single  OutDataType=sfix(16)  OutScaling=2^0  OutDataTypeStr=single
  IncrementRate : Stateflow chart  TreatAsAtomicUnit=on
  PulseTime : Constant  Value=10  OutDataTypeMode=single  OutDataType=fixdt(1, 16)  OutScaling=2^0  OutDataTypeStr=single
  WaitIncrement : Constant  Value=1800  OutDataTypeMode=single  OutDataType=fixdt(1, 16)  OutScaling=2^0  OutDataTypeStr=single
  simstep : Constant  Tag=R12-1  Value=SimStep_dT  OutDataTypeMode=double  OutDataType=sfix(16)  OutScaling=2^0  OutDataTypeStr=double
  Profile_Data_inc : Outport  OutDataType=sfix(16)  OutScaling=2^0
  Mode_Cntrl_inc : Outport  Port=2  OutDataType=sfix(16)  OutScaling=2^0
  IncrementStep : Outport  Port=3  OutDataType=sfix(16)  OutScaling=2^0
  wires:
  PulseTime/1 -> IncrementRate/2(PTime)
  IncrementRate/3(Step) -> IncrementStep/1
  IncrementRate/2(Mode_Cntrl) -> Mode_Cntrl_inc/1
  IncrementRate/1(Control_Value) -> Profile_Data_inc/1
  PackVolt_MinCell/1 -> [PackVolt_MinCell]
  Voltage/1 -> [Voltage]
  simstep/1 -> Data Type Conversion1/1
  Data Type Conversion1/1 -> IncrementRate/1(sim_step_time)
  Data Store Read1/1 -> IncrementRate/5(Pulse)
  Data Store Read2/1 -> IncrementRate/6(Increment)
  Data Store Read3/1 -> IncrementRate/7(deltaAhr)
  WaitIncrement/1 -> IncrementRate/8(WaitTime)
  [Voltage] -> IncrementRate/3(Voltage)
  [PackVolt_MinCell] -> IncrementRate/4(PackVolt_MinCell)
  Data Store Read4/1 -> IncrementRate/9(Ahr)
  Data Store Read5/1 -> IncrementRate/10(Vfloor)
  Data Store Read6/1 -> IncrementRate/11(VfloorCell)
  Data Store Read10/1 -> IncrementRate/12(DschrgCal)
  IncrementRate/4(DschrgLimit) -> Data Store Write1/1

== system HIL_Testing_SW/LionsHeart/FeaturePresentation/Down_to_Business/DriveProfile_ModeControl/OCV Test ==
  Current : Inport  OutDataType=fixdt(1, 16)  OutScaling=2^0
  Voltage : Inport  Port=2  OutDataType=fixdt(1, 16)  OutScaling=2^0
  Enable : EnablePort  StatesWhenEnabling=reset
  ChargeRate : Constant  OutDataTypeMode=single  OutDataType=fixdt(1, 16)  OutScaling=2^0  OutDataTypeStr=single
  Data Store Read : DataStoreRead  DataStoreName=Voltage_Floor  SampleTime=0
  Data Store Read1 : DataStoreRead  DataStoreName=Voltage_Lid  SampleTime=0
  Data Store Read10 : DataStoreRead  DataStoreName=DschrgCurrLim  SampleTime=0
  Data Store Read2 : DataStoreRead  DataStoreName=TerminationCurrent  SampleTime=0
  Data Store Read3 : DataStoreRead  DataStoreName=OCVRate  SampleTime=0
  Data Store Read4 : DataStoreRead  DataStoreName=OCVRate  SampleTime=0
  Data Store Read5 : DataStoreRead  DataStoreName=Ahr  SampleTime=0
  Data Store Read6 : DataStoreRead  DataStoreName=OCVRest  SampleTime=0
  Data Store Read7 : DataStoreRead  DataStoreName=deltaAhr  SampleTime=0
  Data Store Read9 : DataStoreRead  DataStoreName=ChrgCurrLim  SampleTime=0
  Data Store Write1 : DataStoreWrite  DataStoreName=ChrgCurrLim  SampleTime=-1
  Data Store Write2 : DataStoreWrite  DataStoreName=DschrgCurrLim  SampleTime=-1
  Data Type Conversion : DataTypeConversion  OutDataTypeMode=single  OutDataType=sfix(16)  OutScaling=2^0  OutDataTypeStr=single
  Data Type Conversion1 : DataTypeConversion  OutDataTypeMode=single  OutDataType=sfix(16)  OutScaling=2^0  OutDataTypeStr=single
  Data Type Conversion2 : DataTypeConversion  OutDataTypeMode=single  OutDataType=sfix(16)  OutScaling=2^0  OutDataTypeStr=single
  DischrgRate : Constant  Value=-1  OutDataTypeMode=single  OutDataType=fixdt(1, 16)  OutScaling=2^0  OutDataTypeStr=single
  DischrgRate1 : Constant  Value=-1  OutDataTypeMode=single  OutDataType=fixdt(1, 16)  OutScaling=2^0  OutDataTypeStr=single
  OCV_Test : Stateflow chart  TreatAsAtomicUnit=on
  Product1 : Product  OutDataType=fixdt(1, 16)  OutScaling=2^0  RndMeth=Zero
  Product2 : Product  OutDataType=fixdt(1, 16)  OutScaling=2^0  RndMeth=Zero
  Product3 : Product  OutDataType=fixdt(1, 16)  OutScaling=2^0  RndMeth=Zero
  Terminator2 : Terminator
  TestEnbl : Constant  Value=0  OutDataTypeMode=double  OutDataType=fixdt(1, 16)  OutScaling=2^0  OutDataTypeStr=double
  TestStep : Constant  Value=0  OutDataTypeMode=double  OutDataType=fixdt(1, 16)  OutScaling=2^0  OutDataTypeStr=double
  simstep : Constant  Tag=R12-1  Value=SimStep_dT  OutDataTypeMode=double  OutDataType=sfix(16)  OutScaling=2^0  OutDataTypeStr=double
  Profile_Data_OCV : Outport  OutDataType=sfix(16)  OutScaling=2^0
  Mode_Cntrl_OCV : Outport  Port=2  OutDataType=sfix(16)  OutScaling=2^0
  OCVStep : Outport  Port=3  OutDataType=sfix(16)  OutScaling=2^0
  ResetSOC : Outport  Port=4  OutDataType=sfix(16)  OutScaling=2^0
  ResetRun : Outport  Port=5  OutDataType=sfix(16)  OutScaling=2^0
  wires:
  Current/1 -> [Current]
  Voltage/1 -> [Voltage]
  ChargeRate/1 -> Product2/1
  Data Store Read4/1 -> Data Type Conversion2/1
  Product2/1 -> [ChrgRate]
  DischrgRate/1 -> Product3/1
  Product3/1 -> [DischrgRate]
  [Voltage] -> OCV_Test/6(Voltage)
  [Current] -> OCV_Test/7(Current)
  [ChrgRate] -> OCV_Test/3(RateChrg)
  [DischrgRate] -> OCV_Test/2(RateDischrg)
  Data Store Read1/1 -> OCV_Test/4(Vlid)
  Data Store Read/1 -> OCV_Test/1(Vfloor)
  simstep/1 -> Data Type Conversion1/1
  Data Type Conversion/1 -> Profile_Data_OCV/1
  OCV_Test/3(Mode_Cntrl_cap) -> Mode_Cntrl_OCV/1
  OCV_Test/1(Control_Value_cap) -> Data Type Conversion/1
  Data Type Conversion1/1 -> OCV_Test/8(sim_step_time)
  OCV_Test/2(WaitTime) -> Terminator2/1  "Waitime"
  OCV_Test/7(ResetSOC) -> ResetSOC/1
  Data Store Read2/1 -> OCV_Test/5(CurrentTerm)
  Data Store Read9/1 -> OCV_Test/9(ChrgCurrLim)
  Data Store Read10/1 -> OCV_Test/10(DischrgCurrLim)
  OCV_Test/4(DischrgCurrLim_Tmp) -> Data Store Write2/1
  OCV_Test/5(ChrgCurrLim_Tmp) -> Data Store Write1/1
  OCV_Test/6(Step) -> OCVStep/1
  [PackSens] -> OCV_Test/11(PackSens)
  [OCVRate] -> OCV_Test/12(RateOCVDischrg)
  Data Store Read5/1 -> OCV_Test/13(Ahr)
  Data Store Read6/1 -> OCV_Test/14(RestTime)
  Data Store Read7/1 -> OCV_Test/15(deltaAhr)
  OCV_Test/8(ResetRun) -> ResetRun/1
  TestEnbl/1 -> OCV_Test/16(Test)
  TestStep/1 -> OCV_Test/17(StepTest)
  Data Store Read3/1 -> Product1/1
  DischrgRate1/1 -> Product1/2
  Product1/1 -> [OCVRate]
  Data Type Conversion2/1 -> Product2/2, Product3/2

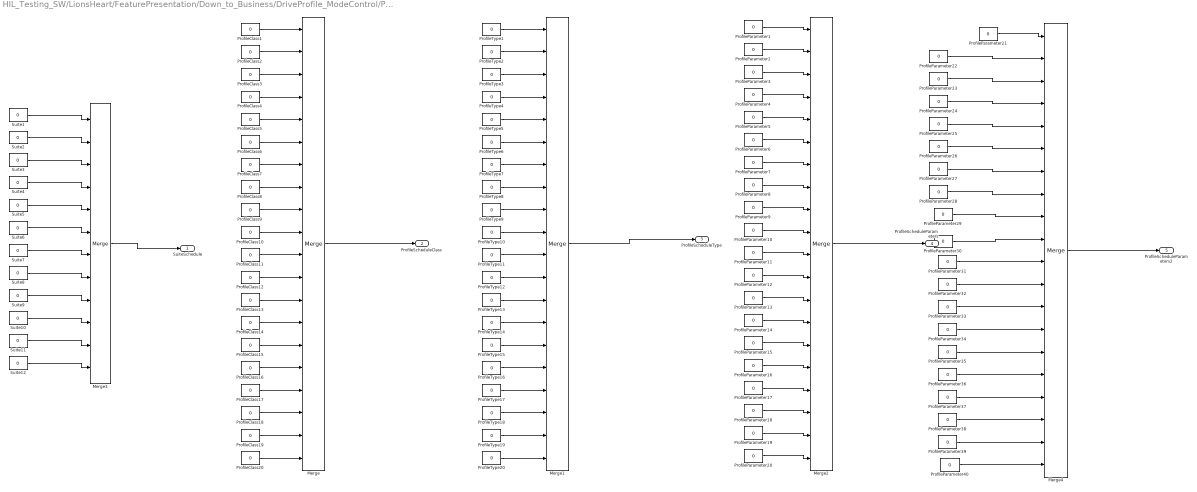
== system HIL_Testing_SW/LionsHeart/FeaturePresentation/Down_to_Business/DriveProfile_ModeControl/ProfileSchedule ==
  Merge{,1..2,4} (4 alike) : Merge  Inputs=20  AllowUnequalInputPortWidths=on  InputPortOffsets=[0 1 2 3 4 5 6 7 8 9 10 11 12 13 14 15 16 17 18 19]
  Merge3 : Merge  Inputs=12  AllowUnequalInputPortWidths=on  InputPortOffsets=[0 1 2 3 4 5 6 7 8 9 10 11]
  ProfileClass{1..20} (20 alike) : Constant  Value=0  VectorParams1D=off  OutDataTypeMode=uint8  OutDataType=Enum: ProfileScheduling  ConRadixGroup=Best Precision: Vector-wise  OutDataTypeStr=uint8
  ProfileParameter{1..40} (40 alike) : Constant  Value=0  VectorParams1D=off  OutDataTypeMode=double  OutDataType=Enum: ProfileScheduling  ConRadixGroup=Best Precision: Vector-wise  OutDataTypeStr=double
  ProfileType{1..20} (20 alike) : Constant  Value=0  VectorParams1D=off  OutDataTypeMode=uint8  OutDataType=Enum: ProfileScheduling  ConRadixGroup=Best Precision: Vector-wise  OutDataTypeStr=uint8
  Suite{1..12} (12 alike) : Constant  Value=0  VectorParams1D=off  OutDataTypeMode=uint8  OutDataType=Enum: ProfileScheduling  ConRadixGroup=Best Precision: Vector-wise  OutDataTypeStr=uint8
  SuiteSchedule : Outport  OutDataType=fixdt(1, 16)  OutScaling=2^0
  ProfileScheduleClass : Outport  Port=2  OutDataType=fixdt(1, 16)  OutScaling=2^0
  ProfileScheduleType : Outport  Port=3  OutDataType=fixdt(1, 16)  OutScaling=2^0
  ProfileScheduleParameters : Outport  Port=4  OutDataType=fixdt(1, 16)  OutScaling=2^0
  ProfileScheduleParameters2 : Outport  Port=5  OutDataType=fixdt(1, 16)  OutScaling=2^0
  wires:
  ProfileClass1/1 -> Merge/1
  ProfileClass2/1 -> Merge/2
  ProfileClass3/1 -> Merge/3
  ProfileClass4/1 -> Merge/4
  ProfileClass5/1 -> Merge/5
  ProfileClass6/1 -> Merge/6
  ProfileClass7/1 -> Merge/7
  ProfileClass8/1 -> Merge/8
  ProfileClass9/1 -> Merge/9
  ProfileClass10/1 -> Merge/10
  ProfileClass12/1 -> Merge/12
  ProfileClass11/1 -> Merge/11
  ProfileClass13/1 -> Merge/13
  ProfileClass14/1 -> Merge/14
  ProfileClass15/1 -> Merge/15
  ProfileClass16/1 -> Merge/16
  ProfileClass17/1 -> Merge/17
  ProfileClass18/1 -> Merge/18
  ProfileClass19/1 -> Merge/19
  ProfileClass20/1 -> Merge/20
  ProfileType1/1 -> Merge1/1
  ProfileType2/1 -> Merge1/2
  ProfileType3/1 -> Merge1/3
  ProfileType4/1 -> Merge1/4
  ProfileType5/1 -> Merge1/5
  ProfileType6/1 -> Merge1/6
  ProfileType7/1 -> Merge1/7
  ProfileType8/1 -> Merge1/8
  ProfileType9/1 -> Merge1/9
  ProfileType10/1 -> Merge1/10
  ProfileType12/1 -> Merge1/12
  ProfileType11/1 -> Merge1/11
  ProfileType13/1 -> Merge1/13
  ProfileType14/1 -> Merge1/14
  ProfileType15/1 -> Merge1/15
  ProfileType16/1 -> Merge1/16
  ProfileType17/1 -> Merge1/17
  ProfileType18/1 -> Merge1/18
  ProfileType19/1 -> Merge1/19
  ProfileType20/1 -> Merge1/20
  ProfileParameter1/1 -> Merge2/1
  ProfileParameter2/1 -> Merge2/2
  ProfileParameter3/1 -> Merge2/3
  ProfileParameter4/1 -> Merge2/4
  ProfileParameter5/1 -> Merge2/5
  ProfileParameter6/1 -> Merge2/6
  ProfileParameter7/1 -> Merge2/7
  ProfileParameter8/1 -> Merge2/8
  ProfileParameter9/1 -> Merge2/9
  ProfileParameter10/1 -> Merge2/10
  ProfileParameter12/1 -> Merge2/12
  ProfileParameter11/1 -> Merge2/11
  ProfileParameter13/1 -> Merge2/13
  ProfileParameter14/1 -> Merge2/14
  ProfileParameter15/1 -> Merge2/15
  ProfileParameter16/1 -> Merge2/16
  ProfileParameter17/1 -> Merge2/17
  ProfileParameter18/1 -> Merge2/18
  ProfileParameter19/1 -> Merge2/19
  ProfileParameter20/1 -> Merge2/20
  Suite1/1 -> Merge3/1
  Suite2/1 -> Merge3/2
  Suite3/1 -> Merge3/3
  Suite4/1 -> Merge3/4
  Suite5/1 -> Merge3/5
  Suite6/1 -> Merge3/6
  Suite7/1 -> Merge3/7
  Suite8/1 -> Merge3/8
  Suite9/1 -> Merge3/9
  Suite10/1 -> Merge3/10
  Suite12/1 -> Merge3/12
  Suite11/1 -> Merge3/11
  Merge3/1 -> SuiteSchedule/1
  Merge/1 -> ProfileScheduleClass/1
  Merge1/1 -> ProfileScheduleType/1
  Merge2/1 -> ProfileScheduleParameters/1
  ProfileParameter21/1 -> Merge4/1
  Merge4/1 -> ProfileScheduleParameters2/1
  ProfileParameter40/1 -> Merge4/20
  ProfileParameter39/1 -> Merge4/19
  ProfileParameter38/1 -> Merge4/18
  ProfileParameter37/1 -> Merge4/17
  ProfileParameter36/1 -> Merge4/16
  ProfileParameter35/1 -> Merge4/15
  ProfileParameter34/1 -> Merge4/14
  ProfileParameter33/1 -> Merge4/13
  ProfileParameter32/1 -> Merge4/12
  ProfileParameter31/1 -> Merge4/11
  ProfileParameter30/1 -> Merge4/10
  ProfileParameter29/1 -> Merge4/9
  ProfileParameter28/1 -> Merge4/8
  ProfileParameter27/1 -> Merge4/7
  ProfileParameter26/1 -> Merge4/6
  ProfileParameter25/1 -> Merge4/5
  ProfileParameter24/1 -> Merge4/4
  ProfileParameter23/1 -> Merge4/3
  ProfileParameter22/1 -> Merge4/2

== system HIL_Testing_SW/LionsHeart/FeaturePresentation/Down_to_Business/DriveProfile_ModeControl/ProfileScheduleBreakout ==
  Class : Inport  OutDataType=fixdt(1, 16)  OutScaling=2^0
  Type : Inport  Port=2  OutDataType=fixdt(1, 16)  OutScaling=2^0
  Parameter : Inport  Port=3  OutDataType=fixdt(1, 16)  OutScaling=2^0
  Step : Inport  Port=4  OutDataType=fixdt(1, 16)  OutScaling=2^0
  Class Breakout : Stateflow chart  TreatAsAtomicUnit=on
  Multiport Switch : MultiPortSwitch  Inputs=20  zeroidx=off  OutDataType=fixdt(1, 16)  OutScaling=2^0
  Multiport Switch1 : MultiPortSwitch  Inputs=20  zeroidx=off  OutDataType=fixdt(1, 16)  OutScaling=2^0
  Parameter Breakout : Stateflow chart  TreatAsAtomicUnit=on
  Terminator{40..59} (20 alike) : Terminator
  Type Breakout : Stateflow chart  TreatAsAtomicUnit=on
  ActiveClass : Outport  OutDataType=fixdt(1, 16)  OutScaling=2^0
  ActiveType : Outport  Port=2  OutDataType=fixdt(1, 16)  OutScaling=2^0
  wires:
  Class/1 -> Class Breakout/1(list)
  Class Breakout/1(item1) -> Multiport Switch/2
  Class Breakout/2(item2) -> Multiport Switch/3
  Class Breakout/3(item3) -> Multiport Switch/4
  Class Breakout/5(item5) -> Multiport Switch/6
  Class Breakout/6(item6) -> Multiport Switch/7
  Class Breakout/7(item7) -> Multiport Switch/8
  Class Breakout/9(item9) -> Multiport Switch/10
  Class Breakout/10(item10) -> Multiport Switch/11
  Class Breakout/11(item11) -> Multiport Switch/12
  Class Breakout/12(item12) -> Multiport Switch/13
  Class Breakout/13(item13) -> Multiport Switch/14
  Class Breakout/14(item14) -> Multiport Switch/15
  Class Breakout/15(item15) -> Multiport Switch/16
  Class Breakout/16(item16) -> Multiport Switch/17
  Class Breakout/17(item17) -> Multiport Switch/18
  Class Breakout/18(item18) -> Multiport Switch/19
  Class Breakout/19(item19) -> Multiport Switch/20
  Class Breakout/20(item20) -> Multiport Switch/21
  Type Breakout/1(item1) -> Multiport Switch1/2
  Type Breakout/2(item2) -> Multiport Switch1/3
  Type Breakout/3(item3) -> Multiport Switch1/4
  Type Breakout/5(item5) -> Multiport Switch1/6
  Type Breakout/6(item6) -> Multiport Switch1/7
  Type Breakout/7(item7) -> Multiport Switch1/8
  Type Breakout/8(item8) -> Multiport Switch1/9
  Type Breakout/9(item9) -> Multiport Switch1/10
  Type Breakout/10(item10) -> Multiport Switch1/11
  Type Breakout/11(item11) -> Multiport Switch1/12
  Type Breakout/12(item12) -> Multiport Switch1/13
  Type Breakout/13(item13) -> Multiport Switch1/14
  Type Breakout/14(item14) -> Multiport Switch1/15
  Type Breakout/15(item15) -> Multiport Switch1/16
  Type Breakout/17(item17) -> Multiport Switch1/18
  Type Breakout/18(item18) -> Multiport Switch1/19
  Type Breakout/19(item19) -> Multiport Switch1/20
  Type Breakout/20(item20) -> Multiport Switch1/21
  Type/1 -> Type Breakout/1(list)
  Parameter Breakout/1(item1) -> Terminator40/1
  Parameter Breakout/2(item2) -> Terminator41/1
  Parameter Breakout/3(item3) -> Terminator52/1
  Parameter Breakout/4(item4) -> Terminator53/1
  Parameter Breakout/5(item5) -> Terminator54/1
  Parameter Breakout/6(item6) -> Terminator55/1
  Parameter Breakout/7(item7) -> Terminator56/1
  Parameter Breakout/8(item8) -> Terminator57/1
  Parameter Breakout/9(item9) -> Terminator58/1
  Parameter Breakout/10(item10) -> Terminator59/1
  Parameter Breakout/11(item11) -> Terminator42/1
  Parameter Breakout/12(item12) -> Terminator43/1
  Parameter Breakout/13(item13) -> Terminator44/1
  Parameter Breakout/14(item14) -> Terminator45/1
  Parameter Breakout/15(item15) -> Terminator46/1
  Parameter Breakout/16(item16) -> Terminator47/1
  Parameter Breakout/17(item17) -> Terminator48/1
  Parameter Breakout/18(item18) -> Terminator49/1
  Parameter Breakout/19(item19) -> Terminator50/1
  Parameter Breakout/20(item20) -> Terminator51/1
  Parameter/1 -> Parameter Breakout/1(list)
  Step/1 -> [Step]
  Class Breakout/4(item4) -> Multiport Switch/5
  Class Breakout/8(item8) -> Multiport Switch/9
  [Step] -> Multiport Switch/1
  Multiport Switch/1 -> ActiveClass/1
  Multiport Switch1/1 -> ActiveType/1
  [Step] -> Multiport Switch1/1
  Type Breakout/4(item4) -> Multiport Switch1/5
  Type Breakout/16(item16) -> Multiport Switch1/17
